simulink model "untitled"  (R2017b)
settings: Solver=FixedStepDiscrete  StartTime=0.0  StopTime=20  FixedStep=dt  RelTol=1e-3
values from neighbouring files (symbols this model uses):
  dt = 0.1    [extendedKalmanFilter.m]    (also in matlab.mat; runV3.m; rungen.m; runpathfollower.m)
  xi0 = [0 0 0 0 0 0 0 0]    [matlab.mat]    (also in runV3.m = [0 0 0 0 0 0 0 0]'; runpathfollower.m = [xi,yi,0,0,0,0,theta_mi,0]'; runpathplanner.m = [xi,yi,0,0,0,0,theta_mi,0]')
libraries: simulink x3
settings Model: Creator=nisha  LastModifiedBy=nisha

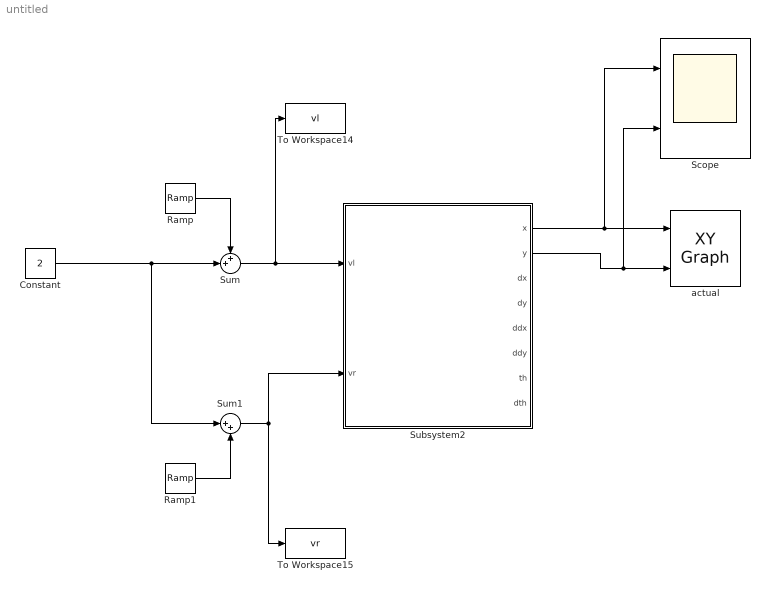
== system untitled ==
  Constant : Constant  Value=2
  Ramp : simulink/Sources/Ramp  slope=0.1  start=2  X0=0
  Ramp1 : simulink/Sources/Ramp  slope=0.1  start=3  X0=0
  Scope : Scope  NumInputPorts=2
  Subsystem2 : Subsystem
  Sum : Sum  Inputs=++|
  Sum1 : Sum  Inputs=|++
  To Workspace14 : ToWorkspace  VariableName=vl  SampleTime=-1
  To Workspace15 : ToWorkspace  VariableName=vr  SampleTime=-1
  actual : simulink/Sinks/XY Graph  xmin=-5  xmax=50  ymin=-15  ymax=50  st=-1
  wires:
  Ramp1/1 -> Sum1/2
  Sum1/1 -> Subsystem2/2(vr), To Workspace15/1
  Constant/1 -> Sum1/1, Sum/2
  Ramp/1 -> Sum/1
  Sum/1 -> Subsystem2/1(vl), To Workspace14/1
  Subsystem2/1(x) -> Scope/1, actual/1
  Subsystem2/2(y) -> Scope/2, actual/2

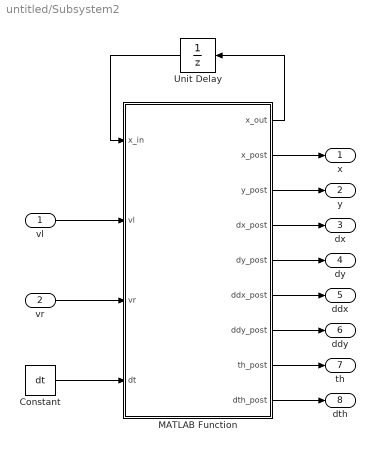
== system untitled/Subsystem2 ==
  vl : Inport
  vr : Inport  Port=2
  Constant : Constant  Value=dt
  MATLAB Function : MATLAB Function  TreatAsAtomicUnit=on
  Unit Delay : UnitDelay  InitialCondition=xi0  SampleTime=-1
  x : Outport
  y : Outport  Port=2
  dx : Outport  Port=3
  dy : Outport  Port=4
  ddx : Outport  Port=5
  ddy : Outport  Port=6
  th : Outport  Port=7
  dth : Outport  Port=8
  wires:
  vl/1 -> MATLAB Function/2(vl)
  MATLAB Function/1(x_out) -> Unit Delay/1
  Unit Delay/1 -> MATLAB Function/1(x_in)
  vr/1 -> MATLAB Function/3(vr)
  MATLAB Function/2(x_post) -> x/1
  MATLAB Function/3(y_post) -> y/1
  MATLAB Function/4(dx_post) -> dx/1
  MATLAB Function/5(dy_post) -> dy/1
  MATLAB Function/6(ddx_post) -> ddx/1
  MATLAB Function/7(ddy_post) -> ddy/1
  MATLAB Function/8(th_post) -> th/1
  MATLAB Function/9(dth_post) -> dth/1
  Constant/1 -> MATLAB Function/4(dt)

== matlab function untitled/Subsystem2/MATLAB Function ==
  data: x_in input; x_out output; vl input; vr input; x_post output; y_post output; dx_post output; dy_post output; ddx_post output; ddy_post output; th_post output; dth_post output; dt input
function [x_out,x_post,y_post,dx_post,dy_post,ddx_post,ddy_post,th_post,dth_post]         = fcn(x_in,vl, vr,dt)

d=0.15;
x=x_in(1); y=x_in(2); dx=x_in(3); dy=x_in(4);
ddx=x_in(5); ddy=x_in(6); phi=x_in(7); dphi=x_in(8); 

x_out = ...
[x + dt*dx + (ddx*dt^2)/2 + (dt*vl*cosd(phi))/2 + (dt*vr*cosd(phi))/2
 y + dt*dy + (ddy*dt^2)/2 + (dt*vl*sind(phi))/2 + (dt*vr*sind(phi))/2
                    dx + ddx*dt + (vl*cosd(phi))/2 + (vr*cosd(phi))/2
                    dy + ddy*dt + (vl*sind(phi))/2 + (vr*sind(phi))/2
                                                                ddx
                                                                ddy
                              (d*phi - dt*vl + dt*vr + d*dphi*dt)/d
                                               (vr - vl + d*dphi)/d];

x_post=x_out(1); y_post=x_out(2);dx_post=x_out(3);dy_post=x_out(4);
ddx_post=x_out(5);ddy_post=x_out(6);th_post=x_out(7);dth_post=x_out(8);
end
